simulink model "Punto2"  (R2017b)
settings: Solver=VariableStepAuto  StartTime=0.0  StopTime=.02  RelTol=1e-3
values from neighbouring files (symbols this model uses):
  dc = [.0000001 .0001 1]    [Practica2Control3.m]
  nc = 1    [Practica2Control3.m]
  T1 = .0005    (= 0.0005)    [Practica2Control3.m]
  T2 = .002    (= 0.002)    [Practica2Control3.m]
undefined symbols (not defined in the file or in its folder): dd, dd2, nd, nd2
settings Model: Creator=Agustin  LastModifiedBy=Agustin

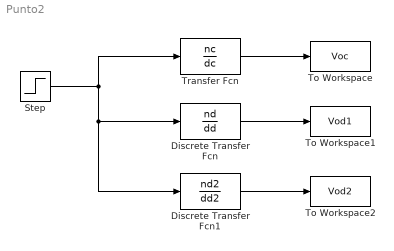
== system Punto2 ==
  Discrete Transfer Fcn : DiscreteTransferFcn  Numerator=nd  Denominator=dd  SampleTime=T1
  Discrete Transfer Fcn1 : DiscreteTransferFcn  Numerator=nd2  Denominator=dd2  SampleTime=T2
  Step : Step  Time=0  SampleTime=0
  To Workspace : ToWorkspace  VariableName=Voc  SaveFormat=Timeseries  SampleTime=-1
  To Workspace1 : ToWorkspace  VariableName=Vod1  SaveFormat=Timeseries  SampleTime=-1
  To Workspace2 : ToWorkspace  VariableName=Vod2  SaveFormat=Timeseries  SampleTime=-1
  Transfer Fcn : TransferFcn  Numerator=nc  Denominator=dc
  wires:
  Transfer Fcn/1 -> To Workspace/1
  Discrete Transfer Fcn/1 -> To Workspace1/1
  Step/1 -> Discrete Transfer Fcn1/1, Discrete Transfer Fcn/1, Transfer Fcn/1
  Discrete Transfer Fcn1/1 -> To Workspace2/1
